simulink model "MoHinhTWB"  (R2022b)
settings: Solver=ode45  StartTime=0.0  StopTime=50  RelTol=1e-3
undefined symbols (not defined in the file): g, Ip, Iw, ke, km, l, Mp, Mw, R, r
settings Model: Creator=buile  LastModifiedBy=Admins
settings SolverCC: AlgebraicLoopSolver=TrustRegion
settings DebuggingCC: UnconnectedInputMsg=warning  UnconnectedOutputMsg=warning  UnconnectedLineMsg=warning  SFMachineParentedDataDiag=warning
settings ModelReferenceCC: EnableRefExpFcnMdlSchedulingChecks=on
settings SFSimCC: CustomCodeUndefinedFunction=UseInterfaceOnly

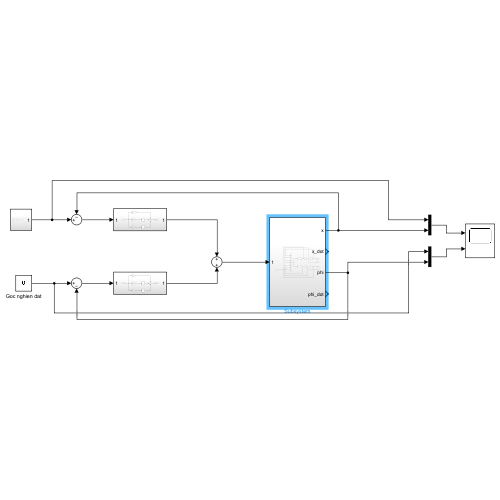
[thumbnail: Simulink's stored preview of the top-level diagram]
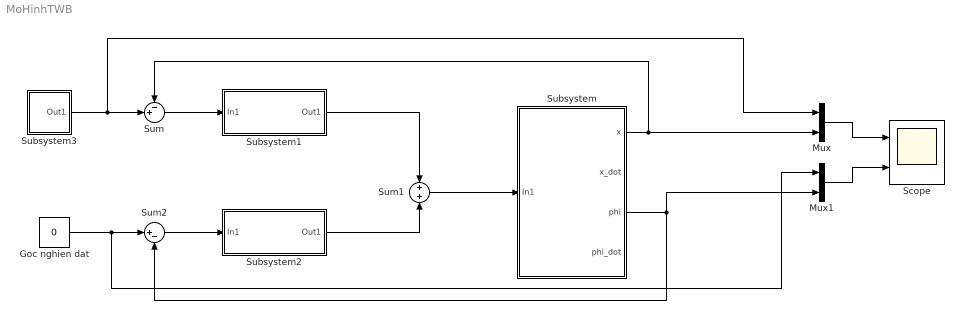
== system MoHinhTWB ==
  Goc nghien dat : Constant  Value=0
  Mux : Mux  Inputs=2
  Mux1 : Mux  Inputs=2
  Scope : Scope  NumInputPorts=2
  Subsystem : Subsystem
  Subsystem1 : Subsystem
  Subsystem2 : Subsystem
  Subsystem3 : Subsystem
  Sum : Sum  Inputs=-+|
  Sum1 : Sum
  Sum2 : Sum  Inputs=|+-
  wires:
  Sum/1 -> Subsystem1/1(In1)
  Subsystem3/1(Out1) -> Mux/1, Sum/2
  Subsystem1/1(Out1) -> Sum1/1
  Subsystem2/1(Out1) -> Sum1/2
  Sum2/1 -> Subsystem2/1(In1)
  Goc nghien dat/1 -> Mux1/1, Sum2/1
  Sum1/1 -> Subsystem/1(In1)
  Subsystem/1(x) -> Sum/1, Mux/2
  Subsystem/3(phi) -> Sum2/2, Mux1/2
  Mux/1 -> Scope/1
  Mux1/1 -> Scope/2

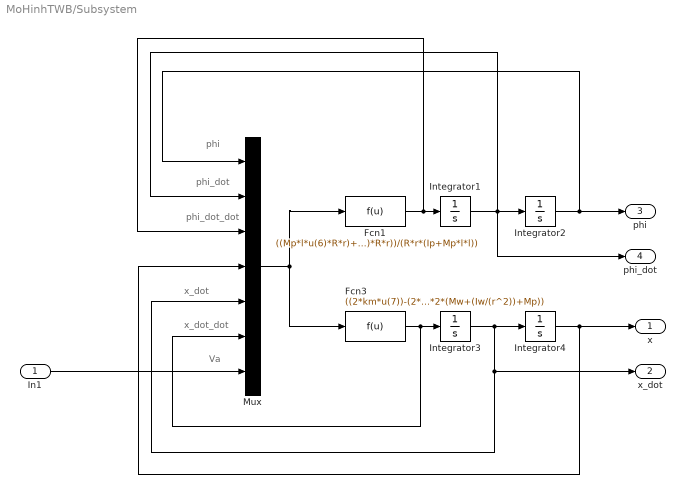
== system MoHinhTWB/Subsystem ==
  note: x_dot_dot
  note: Va
  note: phi
  note: phi_dot_dot
  note: phi_dot
  note: x_dot
  In1 : Inport
  Fcn1 : Fcn  Expr=((Mp*l*u(6)*R*r)+(2*km*ke*u(5))+(2*km*u(7)*r)-(Mp*g*l*u(1)*R*r))/(R*r*(Ip+Mp*l*l))
  Fcn3 : Fcn  Expr=((2*km*u(7))-(2*km*ke*u(5))-(Mp*l*u(3)*R*r))/(R*r*2*(Mw+(Iw/(r^2))+Mp))
  Integrator{1..4} (4 alike) : Integrator
  Mux : Mux  Inputs=7
  x : Outport  VectorParamsAs1DForOutWhenUnconnected=off
  x_dot : Outport  Port=2  VectorParamsAs1DForOutWhenUnconnected=off
  phi : Outport  Port=3  VectorParamsAs1DForOutWhenUnconnected=off
  phi_dot : Outport  Port=4  VectorParamsAs1DForOutWhenUnconnected=off
  wires:
  Fcn3/1 -> Mux/6, Integrator3/1
  Fcn1/1 -> Mux/3, Integrator1/1
  Integrator3/1 -> x_dot/1, Mux/5, Integrator4/1
  Mux/1 -> Fcn1/1, Fcn3/1
  Integrator2/1 -> phi/1, Mux/1
  Integrator1/1 -> phi_dot/1, Mux/2, Integrator2/1
  Integrator4/1 -> x/1, Mux/4
  In1/1 -> Mux/7

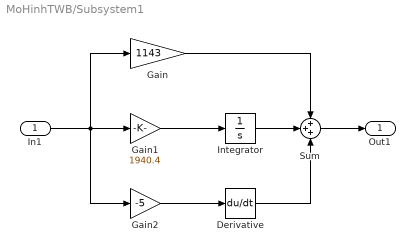
== system MoHinhTWB/Subsystem1 ==
  In1 : Inport
  Derivative : Derivative
  Gain : Gain  Gain=1143
  Gain1 : Gain  Gain=1940.4
  Gain2 : Gain  Gain=-5
  Integrator : Integrator
  Sum : Sum  Inputs=+++
  Out1 : Outport  VectorParamsAs1DForOutWhenUnconnected=off
  wires:
  In1/1 -> Gain2/1, Gain1/1, Gain/1
  Gain1/1 -> Integrator/1
  Gain2/1 -> Derivative/1
  Gain/1 -> Sum/1
  Integrator/1 -> Sum/2
  Derivative/1 -> Sum/3
  Sum/1 -> Out1/1

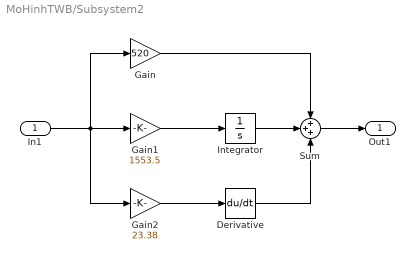
== system MoHinhTWB/Subsystem2 ==
  In1 : Inport
  Derivative : Derivative
  Gain : Gain  Gain=520
  Gain1 : Gain  Gain=1553.5
  Gain2 : Gain  Gain=23.38
  Integrator : Integrator
  Sum : Sum  Inputs=+++
  Out1 : Outport  VectorParamsAs1DForOutWhenUnconnected=off
  wires:
  In1/1 -> Gain2/1, Gain1/1, Gain/1
  Gain1/1 -> Integrator/1
  Gain2/1 -> Derivative/1
  Gain/1 -> Sum/1
  Integrator/1 -> Sum/2
  Derivative/1 -> Sum/3
  Sum/1 -> Out1/1

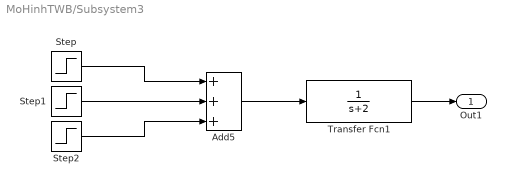
== system MoHinhTWB/Subsystem3 ==
  Add5 : Sum  Inputs=+++
  Step : Step  Time=0  After=0.3  SampleTime=0
  Step1 : Step  Time=20  After=-0.4  SampleTime=0
  Step2 : Step  Time=35  After=0.3  SampleTime=0
  Transfer Fcn1 : TransferFcn  Denominator=[1 2]
  Out1 : Outport
  wires:
  Add5/1 -> Transfer Fcn1/1
  Step1/1 -> Add5/2
  Step/1 -> Add5/1
  Step2/1 -> Add5/3
  Transfer Fcn1/1 -> Out1/1
